simulink model "qnd_sweptsine_1"  (R2021b)
settings: Solver=VariableStepAuto  StartTime=0.0  StopTime=length(foi)*N/Fs + N/Fs  RelTol=1e-3
PreLoadFcn:
  | preload_fcn
values from neighbouring files (symbols this model uses):
  BW = 10e3    (= 10000)    [preload_fcn.m]
  dF = 50    [preload_fcn.m]
  f1 = 100    [preload_fcn.m]
  Fs = OSR*BW    (= 102400)    [preload_fcn.m]
  H = tf([1 0 (2*pi*1e3)^2],[1 2*pi*1e3 (2*pi*1e3)^2])    [preload_fcn.m]
  N = 4*1024    (= 4096)    [preload_fcn.m]
libraries: dspsrcs4 x4, dspstat3 x2, dspmathops x2, dsparch4 x1
settings Model: SimulationMode=accelerator  NumberOfSteps=4096  Creator=kschutz  LastModifiedBy=kschutz

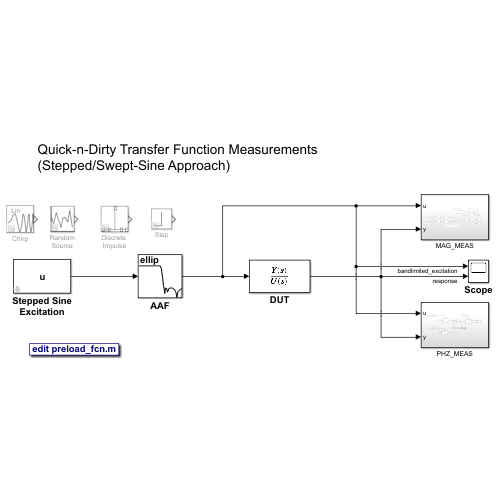
[thumbnail: Simulink's stored preview of the top-level diagram]
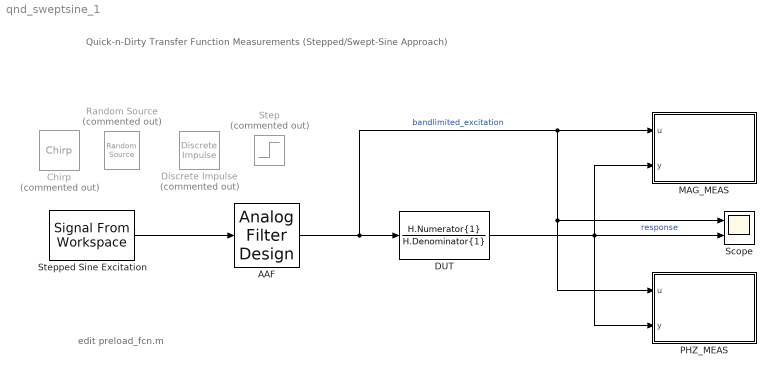
== system qnd_sweptsine_1 ==
  note: edit preload_fcn.m
  note: Quick-n-Dirty Transfer Function Measurements
      | (Stepped/Swept-Sine Approach)
  AAF : dsparch4/Analog Filter Design  method=Elliptic  filttype=Lowpass  N=8  Wlo=2*pi*BW  Whi=80  Rp=.5  Rs=80
  Chirp : dspsrcs4/Chirp  Commented=on  sweep=Linear  mode=Unidirectional  f0=1000  f1=4000  t1=1  Tsweep=1  phase=0  Ts=1/8000  spf=1  datatype=Double  OutputFrames=off
  DUT : TransferFcn  Numerator=H.Numerator{1}  Denominator=H.Denominator{1}
  Discrete Impulse : dspsrcs4/Discrete  Impulse  Commented=on  Delay=0  SampleTime=1  FrameSample=1  OutputFrames=off  dataType=double  isSigned=on  wordLen=16  udDataType=sfix(16)  fracBitsMode=Best precision  numFracBits=15  OutDataTypeStr=double  LastOutDataTypeStr=double
  MAG_MEAS : Subsystem
  PHZ_MEAS : Subsystem
  Random Source : dspsrcs4/Random Source  Commented=on  SrcType=Uniform  NormMethod=Ziggurat  CltLength=12  MinVal=0  MaxVal=1  MeanVal=0  VarVal=1  RepMode=Not repeatable  rawSeed=1  IsInherit=off  SampMode=Discrete  SampTime=1  SampFrame=1  DataType=Double  OutComplex=Real  OutputFrames=off
  Scope : Scope  NumInputPorts=2
  Step : Step  Commented=on  SampleTime=0
  Stepped Sine Excitation : dspsrcs4/Signal From Workspace  X=u  Ts=1/Fs  nsamps=1  OutputAfterFinalValue=Setting to zero  ignoreOrWarnInputAndFrameLengths=off  OutputFrames=off
  wires:
  Stepped Sine Excitation/1 -> AAF/1
  DUT/1 -> MAG_MEAS/2(y), PHZ_MEAS/2(y), Scope/2  "response"
  AAF/1 -> Scope/1, PHZ_MEAS/1(u), MAG_MEAS/1(u), DUT/1  "bandlimited_excitation"

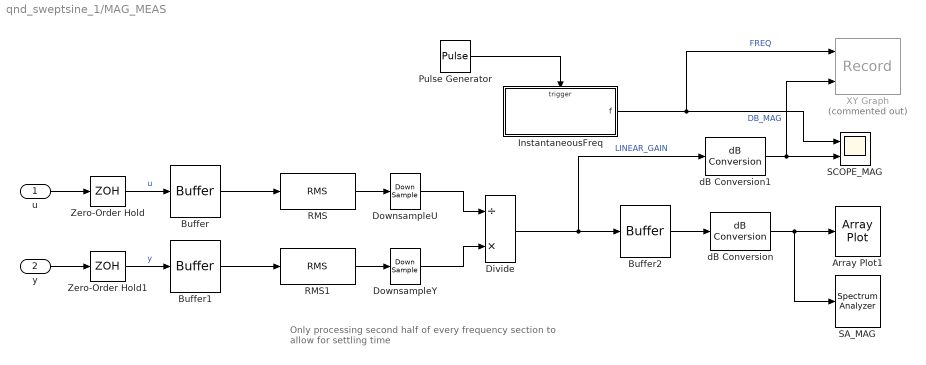
== system qnd_sweptsine_1/MAG_MEAS ==
  note: Only processing second half of every frequency section
      | to allow for settling time
  u : Inport
  y : Inport  Port=2
  Array Plot1 : ArrayPlot  WindowPosition=[1046.000000,599.000000,808.000000,440.000000,]  Visible=on  SampleIncrement=50  XOffset=50  AxesScaling=Manual  YLabel=dB  YLimits=[-50,10]
  Buffer : Buffer  N=N/2  OutputFrames=off
  Buffer1 : Buffer  N=N/2  OutputFrames=off
  Buffer2 : Buffer  N=199  OutputFrames=off
  Divide : Product  Inputs=/*
  DownsampleU : DownSample  phase=1  RateOptions=Allow multirate processing
  DownsampleY : DownSample  phase=1  RateOptions=Allow multirate processing
  InstantaneousFreq : Subsystem
  Pulse Generator : DiscretePulseGenerator  PulseType=Time based  Period=N/Fs  PulseWidth=50
  RMS : dspstat3/RMS  run=off  directionMode=Each column  dimension=1  InputProcessing=Columns as channels (frame based)  reset_popup=None
  RMS1 : dspstat3/RMS  run=off  directionMode=Each column  dimension=1  InputProcessing=Columns as channels (frame based)  reset_popup=None
  SA_MAG : SpectrumAnalyzer  IsFrequencyInputMode=1
  SCOPE_MAG : Scope  NumInputPorts=2
  XY Graph : Record  Commented=on  FileSettingsInternal="{\"entries\":[{\"content\":{\"excelSettings\":{\"content\":{},\"type\":\"Streamout.ExcelSettings\"}},\"type\":\"Streamout.FileSettingStorage\",\"uuid\":\"e7d0fb3e-04ce-438c-9650-b0d56b11f8c1\"}],\"packageUris\":[\"http://schema.mathworks.com/mf0/streamout_blocks/R2020a\"],\"version\":\"1.0\"}"  Layout=[1 1]  SignalsInternal="{\"entries\":[{\"content\":{\"signals\":[]},\"type\":\"RecordBlkView.InputSignals\",\"uuid\":\"58b58989-24ca-49f3-ada3-a26b3d12abcd\"}],\"packageUris\":[\"http://schema.mathworks.com/mf0/streamout_blocks/R2020a\"],\"version\":\"1.0\"}"  VisualizationBindings="{\"xyplotplugin\":{\"info\":[{\"series\":[],\"subplotID\":1}]}}"  CompatibilityTag=XY
  Zero-Order Hold : ZeroOrderHold  SampleTime=1/Fs
  Zero-Order Hold1 : ZeroOrderHold  SampleTime=1/Fs
  dB Conversion : dspmathops/dB Conversion  dBtype=dB  intype=Amplitude  R=1  fuzz=off
  dB Conversion1 : dspmathops/dB Conversion  dBtype=dB  intype=Amplitude  R=1  fuzz=off
  wires:
  Pulse Generator/1 -> InstantaneousFreq/Trigger
  u/1 -> Zero-Order Hold/1
  dB Conversion/1 -> Array Plot1/1, SA_MAG/1
  Buffer2/1 -> dB Conversion/1
  Divide/1 -> dB Conversion1/1, Buffer2/1  "LINEAR_GAIN"
  y/1 -> Zero-Order Hold1/1
  Zero-Order Hold/1 -> Buffer/1  "u"
  Zero-Order Hold1/1 -> Buffer1/1  "y"
  InstantaneousFreq/1(f) -> XY Graph/1, SCOPE_MAG/1  "FREQ"
  dB Conversion1/1 -> XY Graph/2, SCOPE_MAG/2  "DB_MAG"
  Buffer/1 -> RMS/1
  Buffer1/1 -> RMS1/1
  RMS/1 -> DownsampleU/1
  RMS1/1 -> DownsampleY/1
  DownsampleU/1 -> Divide/1
  DownsampleY/1 -> Divide/2

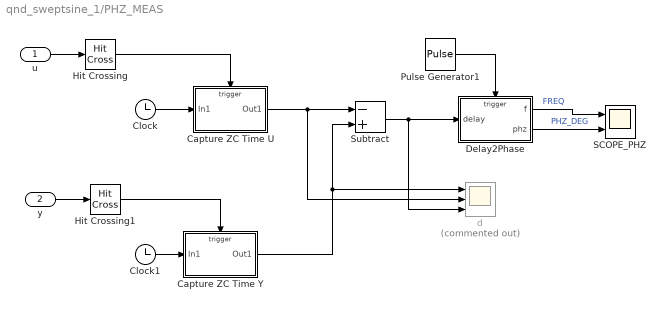
== system qnd_sweptsine_1/PHZ_MEAS ==
  u : Inport
  y : Inport  Port=2
  Capture ZC Time U : Subsystem  TreatAsAtomicUnit=on
  Capture ZC Time Y : Subsystem  TreatAsAtomicUnit=on
  Clock : Clock
  Clock1 : Clock
  Delay2Phase : Subsystem  TreatAsAtomicUnit=on
  Hit Crossing : HitCross  HitCrossingDirection=rising
  Hit Crossing1 : HitCross  HitCrossingDirection=rising
  Pulse Generator1 : DiscretePulseGenerator  PulseType=Time based  Period=N/Fs  PulseWidth=50
  SCOPE_PHZ : Scope  NumInputPorts=2
  Subtract : Sum  Inputs=-+
  d : Scope  Commented=on  NumInputPorts=3
  wires:
  Clock/1 -> Capture ZC Time U/1(In1)
  y/1 -> Hit Crossing1/1
  Pulse Generator1/1 -> Delay2Phase/Trigger
  Clock1/1 -> Capture ZC Time Y/1(In1)
  Subtract/1 -> d/3, Delay2Phase/1(delay)
  Hit Crossing/1 -> Capture ZC Time U/Trigger
  Delay2Phase/2(phz) -> SCOPE_PHZ/2  "PHZ_DEG"
  Hit Crossing1/1 -> Capture ZC Time Y/Trigger
  u/1 -> Hit Crossing/1
  Capture ZC Time U/1(Out1) -> d/2, Subtract/1
  Capture ZC Time Y/1(Out1) -> Subtract/2, d/1
  Delay2Phase/1(f) -> SCOPE_PHZ/1  "FREQ"

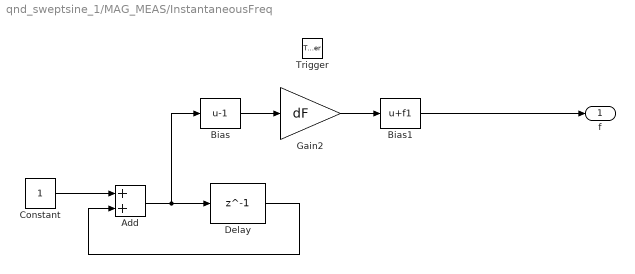
== system qnd_sweptsine_1/MAG_MEAS/InstantaneousFreq ==
  Trigger : TriggerPort  VariantControl=(inherit)  PortDimensions=1
  Add : Sum
  Bias : Bias  Bias=-1
  Bias1 : Bias  Bias=f1
  Constant : Constant
  Delay : Delay  DelayLength=1  InputProcessing=Columns as channels (frame based)
  Gain2 : Gain  Gain=dF
  f : Outport
  wires:
  Add/1 -> Delay/1, Bias/1
  Gain2/1 -> Bias1/1
  Constant/1 -> Add/1
  Delay/1 -> Add/2
  Bias/1 -> Gain2/1
  Bias1/1 -> f/1

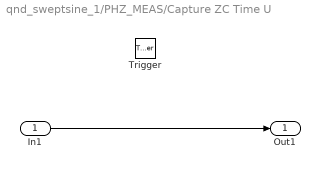
== system qnd_sweptsine_1/PHZ_MEAS/Capture ZC Time U ==
  In1 : Inport
  Trigger : TriggerPort  VariantControl=(inherit)
  Out1 : Outport
  wires:
  In1/1 -> Out1/1

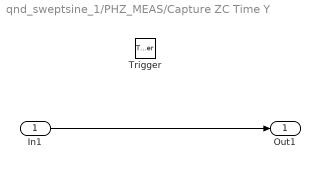
== system qnd_sweptsine_1/PHZ_MEAS/Capture ZC Time Y ==
  In1 : Inport
  Trigger : TriggerPort  VariantControl=(inherit)
  Out1 : Outport
  wires:
  In1/1 -> Out1/1

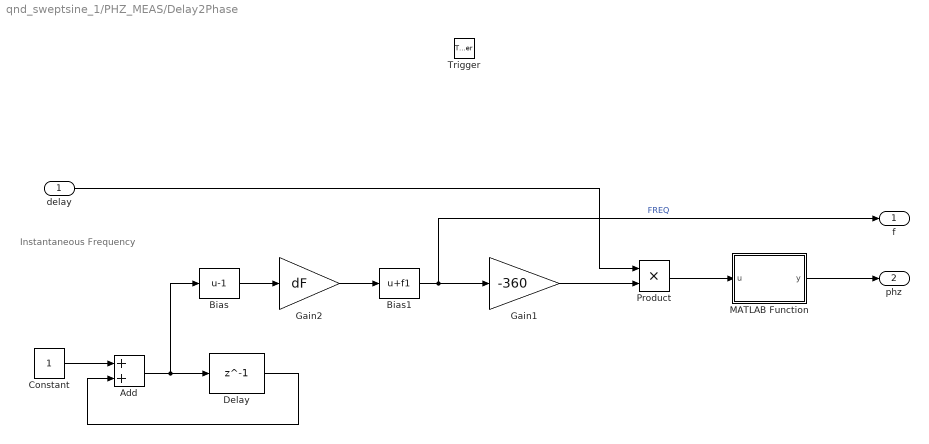
== system qnd_sweptsine_1/PHZ_MEAS/Delay2Phase ==
  note: Instantaneous Frequency
  delay : Inport
  Trigger : TriggerPort  VariantControl=(inherit)
  Add : Sum
  Bias : Bias  Bias=-1
  Bias1 : Bias  Bias=f1
  Constant : Constant
  Delay : Delay  DelayLength=1  InputProcessing=Columns as channels (frame based)
  Gain1 : Gain  Gain=-360
  Gain2 : Gain  Gain=dF
  MATLAB Function : MATLAB Function  TreatAsAtomicUnit=on
  Product : Product
  f : Outport
  phz : Outport  Port=2
  wires:
  delay/1 -> Product/1
  Add/1 -> Delay/1, Bias/1
  Delay/1 -> Add/2
  Constant/1 -> Add/1
  Gain1/1 -> Product/2
  Product/1 -> MATLAB Function/1(u)
  MATLAB Function/1(y) -> phz/1
  Bias/1 -> Gain2/1
  Gain2/1 -> Bias1/1
  Bias1/1 -> Gain1/1, f/1  "FREQ"

== matlab function qnd_sweptsine_1/PHZ_MEAS/Delay2Phase/MATLAB Function ==
  data: u input; y output
function y = wrap180(u)
if u < -180
    y = u + 360;
elseif u > 180
    y = u - 360;
else
    y = u;
end
